simulink model "rob_sim"  (Simulink 7.5)
settings: Solver=ode3  StartTime=0.0  StopTime=1.0  FixedStep=t_step  RelTol=1e-3
undefined symbols (not defined in the file): maxxygraph, rob
libraries: simulink x1
settings Model: Creator=graviton  LastModifiedBy=graviton

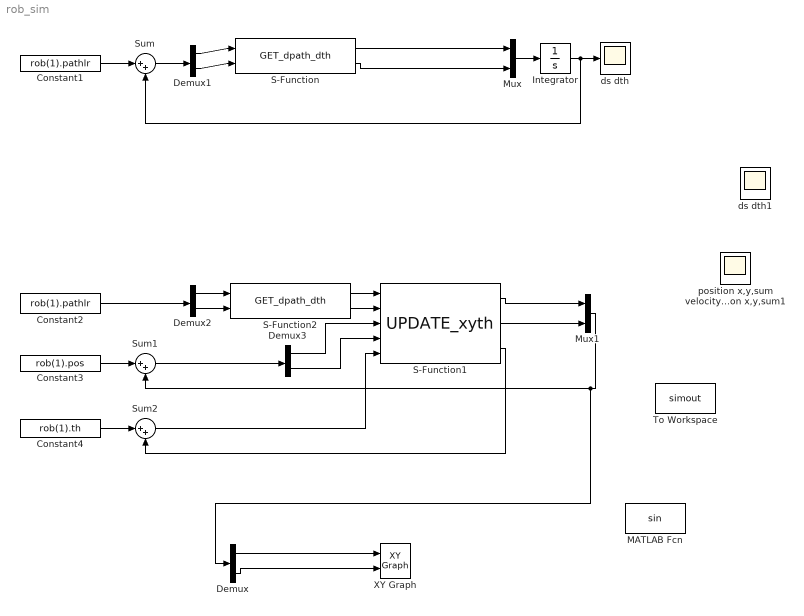
== system rob_sim ==
  Constant1 : Constant  Value=rob(1).pathlr  OutDataType=fixdt(1, 16)  OutScaling=2^0
  Constant2 : Constant  Value=rob(1).pathlr  OutDataType=fixdt(1, 16)  OutScaling=2^0
  Constant3 : Constant  Value=rob(1).pos  OutDataType=fixdt(1, 16)  OutScaling=2^0
  Constant4 : Constant  Value=rob(1).th  OutDataType=fixdt(1, 16)  OutScaling=2^0
  Demux{,1..3} (4 alike) : Demux  Outputs=2
  Integrator : Integrator
  MATLAB Fcn : MATLABFcn
  Mux : Mux  Inputs=2
  Mux1 : Mux  Inputs=2
  S-Function : S-Function  FunctionName=GET_dpath_dth  Parameters=rob(1).base t_step  EnableBusSupport=off
  S-Function1 : S-Function  FunctionName=UPDATE_xyth  Parameters=rob(1).base t_step  EnableBusSupport=off
  S-Function2 : S-Function  FunctionName=GET_dpath_dth  Parameters=rob(1).base t_step  EnableBusSupport=off
  Sum : Sum  Inputs=|++  OutDataType=fixdt(1, 16)  OutScaling=2^0
  Sum1 : Sum  Inputs=|++  OutDataType=fixdt(1, 16)  OutScaling=2^0
  Sum2 : Sum  Inputs=|++  OutDataType=fixdt(1, 16)  OutScaling=2^0
  To Workspace : ToWorkspace  VariableName=simout  SampleTime=-1  SaveFormat=Structure
  XY Graph : simulink/Sinks/XY Graph  SystemSampleTime=-1  xmin=-maxxygraph  xmax=maxxygraph  ymin=-maxxygraph  ymax=maxxygraph  st=-1
  ds dth : Scope
  ds dth1 : Scope
      settings: SaveName=ScopeData2
  position x,y,sum velocity x,y,sum acceleration x,y,sum1 : Scope
  wires:
  Demux/2 -> XY Graph/2
  Demux/1 -> XY Graph/1
  Demux1/1 -> S-Function/1
  Demux1/2 -> S-Function/2
  S-Function/1 -> Mux/1
  S-Function/2 -> Mux/2
  Constant1/1 -> Sum/1
  Sum/1 -> Demux1/1
  Mux/1 -> Integrator/1
  Integrator/1 -> ds dth/1, Sum/2
  S-Function2/1 -> S-Function1/1
  Demux2/1 -> S-Function2/1
  Demux2/2 -> S-Function2/2
  S-Function2/2 -> S-Function1/2
  Constant2/1 -> Demux2/1
  S-Function1/1 -> Mux1/1
  S-Function1/2 -> Mux1/2
  Constant3/1 -> Sum1/1
  Mux1/1 -> Sum1/2, Demux/1
  Sum1/1 -> Demux3/1
  Demux3/1 -> S-Function1/3
  Demux3/2 -> S-Function1/4
  Constant4/1 -> Sum2/1
  S-Function1/3 -> Sum2/2
  Sum2/1 -> S-Function1/5
